simulink model "StepUp Bridge Cycloconverter"  (R2017a)
settings: Solver=ode23s  StartTime=0.0  StopTime=0.04  RelTol=1e-3  EnableMultiTasking=on
libraries: powerlib x13
settings Model: Creator=Femi  LastModifiedBy=sujee
settings DataIOCC: LimitDataPoints=on  SaveFormat=Array  SignalLoggingSaveFormat=ModelDataLogs
settings OptimizationCC: InitFltsAndDblsToZero=on  LifeSpan=inf
settings DebuggingCC: SaveWithParameterizedLinksMsg=none  UnderspecifiedInitializationDetection=Classic  MergeDetectMultiDrivingBlocksExec=none  SignalResolutionControl=TryResolveAllWithWarning  MultiTaskDSMMsg=warning  MultiTaskCondExecSysMsg=none  FcnCallInpInsideContextMsg=warning  SFUnexpectedBacktrackingDiag=warning  SFNoUnconditionalDefaultTransitionDiag=warning  SFExecutionAtInitializationDiag=none
settings HardwareCC: ProdBitPerPointer=32  ProdBitPerSizeT=32  ProdBitPerPtrDiffT=32  ProdLargestAtomicFloat=None  ProdIntDivRoundTo=Undefined  ProdEndianess=Unspecified  ProdWordSize=32  ProdHWDeviceType=32-bit Generic
settings ModelReferenceCC: PropagateSignalLabelsOutOfModel=off
settings SFSimCC: SimUseLocalCustomCode=on
settings RTWCC: RTWUseLocalCustomCode=on
settings GRTTargetCC: TargetFcnLib=ansi_tfl_tmw.mat  TargetLangStandard=C89/C90 (ANSI)  CombineOutputUpdateFcns=off  GRTInterface=on
settings ConfigComp: CovMetricSettings=dw  CovSaveCumulativeToWorkspaceVar=on  CovSaveSingleToWorkspaceVar=on

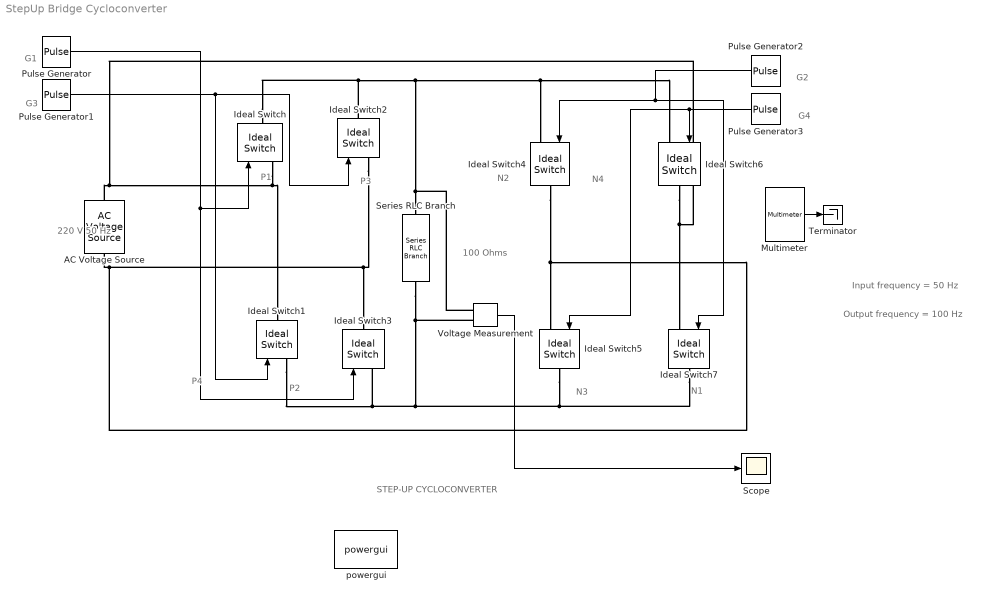
== system StepUp Bridge Cycloconverter ==
  note: P1
  note: P2
  note: P3
  note: P4
  note: N2
  note: N4
  note: N3
  note: N1
  note: 220 V
      | 50 Hz
  note: G1
  note: G3
  note: G2
  note: G4
  note: 100 Ohms
  note: STEP-UP CYCLOCONVERTER
  note: Input frequency = 50 Hz
  note: Output frequency = 100 Hz
  AC Voltage Source : powerlib/Electrical Sources/AC Voltage Source  Amplitude=220  Phase=0  Frequency=50  SampleTime=0  Measurements=Voltage  BusType=swing  Pref=10e3  Qref=0  Qmin=-inf  Qmax=+inf
  Ideal Switch{,1..7} (8 alike) : powerlib/Power Electronics/Ideal Switch  Ron=0.001  Lon=0  IC=0  Rs=1e5  Cs=inf  Measurements=off
  Multimeter : powerlib/Measurements/Multimeter  PhasorSimulation=off  OutputType=Complex  sel=[1 3 2]  L=3  Gain=[1 1 1]  yselected={'Ub: Series RLC Branch','Ib: Series RLC Branch','Usrc: AC Voltage Source'};  PSBOutputType=1  PSBequivalent=0  AxesSetting=[0,0.1,-100,100]  Display=1  SavedBlockNames=-11
  Pulse Generator : DiscretePulseGenerator  PulseType=Time based  Amplitude=5  Period=0.02  PulseWidth=25
  Pulse Generator1 : DiscretePulseGenerator  PulseType=Time based  Amplitude=5  Period=0.02  PulseWidth=25  PhaseDelay=0.01
  Pulse Generator2 : DiscretePulseGenerator  PulseType=Time based  Amplitude=5  Period=0.02  PulseWidth=25  PhaseDelay=0.005
  Pulse Generator3 : DiscretePulseGenerator  PulseType=Time based  Amplitude=5  Period=0.02  PulseWidth=25  PhaseDelay=0.015
  Scope : Scope
  Series RLC Branch : powerlib/Elements/Series RLC Branch  LConnTagsString=__new0  RConnTagsString=__new0  BranchType=RLC  Resistance=100  Inductance=0  SetiL0=off  InitialCurrent=0  Capacitance=inf  Setx0=off  InitialVoltage=0  Measurements=Branch voltage and current
  Terminator : Terminator
  Voltage Measurement : powerlib/Measurements/Voltage Measurement  PhasorSimulation=off  OutputType=Complex  PSBequivalent=0
  powergui : powerlib/powergui  Priority=1  SimulationMode=Continuous  SampleTime=50e-6  frequency=60  Iterations=50  frequencyindice=50  Pbase=100e6  ErrMax=1e-4  UnitsV=kV  UnitsW=MW  buscounter=0  FunctionMessages=off  echomessages=off  EnableUseOfTLC=off  CurrentSourceSwitches=off  DisableSnubberDevices=off  DisableRonSwitches=off  DisableVfSwitches=off  DisplayEquations=off  AutomaticDiscreteSolvers=off  SolverType=Tustin  Interpol=off  ExternalGateDelay=off  methode=off  Ts=100  x0status=blocks  SPID=off  SwTol=0  HookPort=off  NonlinearTolerance=1e-4  nMaxIteration=100  ContinueOnMaxIteration=off  RestoreLinks=warning  ResistiveCurrentMeasurement=off  Frange=[0:2:500]  Ylog=off  Xlog=on  ShowGrid=off  save=off  variable=ZData  structure=0  ZoomFFT=off  StartTime=0.0  cycles=1  DisplayStyle=1  fundamental=60  FreqAxis=off  MaxFrequency=1000  frequencyindicesteady=1  RmsSteady=1  display=off
  wires:
  Multimeter/1 -> Terminator/1
  Pulse Generator/1 -> Ideal Switch/1, Ideal Switch3/1
  Pulse Generator1/1 -> Ideal Switch2/1, Ideal Switch1/1
  Pulse Generator2/1 -> Ideal Switch7/1, Ideal Switch4/1
  Pulse Generator3/1 -> Ideal Switch5/1, Ideal Switch6/1
  Voltage Measurement/1 -> Scope/1
  connections:
  Ideal Switch6/RConn1 -- Ideal Switch/LConn1 -- Ideal Switch1/RConn1 -- AC Voltage Source/RConn1 -- Ideal Switch7/LConn1
  Ideal Switch4/RConn1 -- Ideal Switch2/LConn1 -- Ideal Switch3/RConn1 -- AC Voltage Source/LConn1 -- Ideal Switch5/LConn1
  Ideal Switch1/LConn1 -- Voltage Measurement/LConn2 -- Series RLC Branch/RConn1 -- Ideal Switch7/RConn1 -- Ideal Switch5/RConn1 -- Ideal Switch3/LConn1
  Ideal Switch/RConn1 -- Ideal Switch4/LConn1 -- Ideal Switch6/LConn1 -- Voltage Measurement/LConn1 -- Series RLC Branch/LConn1 -- Ideal Switch2/RConn1
